simulink subsystem "Rotary_Encoder"  (R2020a)
settings: Solver=VariableStepAuto  StartTime=0.0  StopTime=10.0  RelTol=1e-3
settings Model: Creator=Haier  LastModifiedBy=Haier

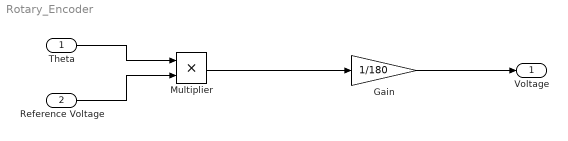
== system Rotary_Encoder ==
  Theta : Inport
  Reference Voltage : Inport  Port=2
  Gain : Gain  Gain=1/180
  Multiplier : Product
  Voltage : Outport  VectorParamsAs1DForOutWhenUnconnected=off
  wires:
  Theta/1 -> Multiplier/1
  Reference Voltage/1 -> Multiplier/2
  Gain/1 -> Voltage/1
  Multiplier/1 -> Gain/1
